simulink model "controle_v1"  (R2025b)
settings: Solver=FixedStepAuto  StartTime=0.0  StopTime=250  RelTol=1e-3
values from neighbouring files (symbols this model uses):
  Ta = 5    [controle_versao1.m]
  tao_1 = 60    [controle_versao1.m]
  tao_2 = 60    [controle_versao1.m]
  w1 = 0    [controle_versao1.m]
  w2 = 0    [controle_versao1.m]
  w3 = 0    [controle_versao1.m]
  w4 = 0    [controle_versao1.m]
undefined symbols (not defined in the file or in its folder): dspblkCoreblockFVToolHelper, gcbh, tao
libraries: dspobslib x1
settings Model: Creator=thoma  LastModifiedBy=thoma
settings ModelReferenceCC: EnableRefExpFcnMdlSchedulingChecks=on
settings RTWCC: GPUComputeCapability=3.5

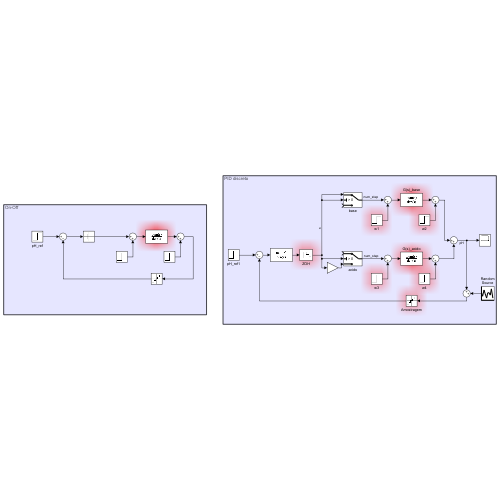
[thumbnail: Simulink's stored preview of the top-level diagram]
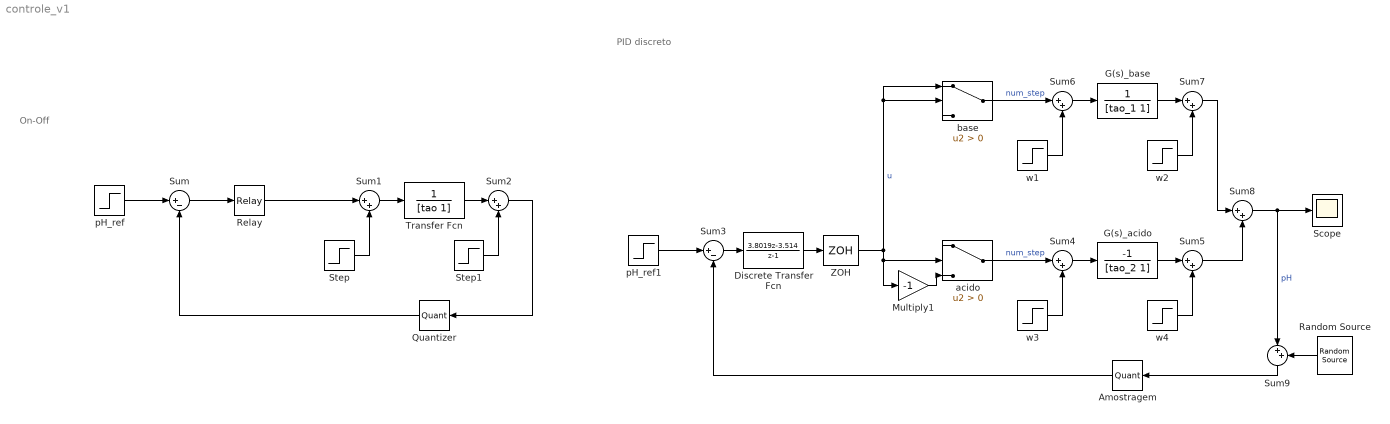
== system controle_v1 ==
  note: PID discreto
  note: On-Off
  Amostragem : Quantizer  QuantizationInterval=Ta
  Discrete Transfer Fcn : DiscreteTransferFcn  LoadFcn=dspblkCoreblockFVToolHelper(gcbh,'load');  Numerator=[3.8019 -3.514]  Denominator=[1 -1]  SampleTime=5
      settings: CopyFcn=dspblkCoreblockFVToolHelper(gcbh,'copy');  DeleteFcn=dspblkCoreblockFVToolHelper(gcbh,'close');  ModelCloseFcn=dspblkCoreblockFVToolHelper(gcbh,'close');  PreSaveFcn=dspblkCoreblockFVToolHelper(gcbh,'presave');  PostSaveFcn=dspblkCoreblockFVToolHelper(gcbh,'postsave');  CloseFcn=dspblkCoreblockFVToolHelper(gcbh,'close');
  G(s)_acido : TransferFcn  Numerator=[-1]  Denominator=[tao_2 1]
  G(s)_base : TransferFcn  Denominator=[tao_1 1]
  Multiply1 : Gain  Gain=-1
  Quantizer : Quantizer
  Random Source : dspobslib/Random Source  SrcType=Gaussian  NormMethod=Ziggurat  CltLength=12  MinVal=0  MaxVal=1  MeanVal=0  VarVal=1  RepMode=Not repeatable  rawSeed=1  IsInherit=off  SampMode=Continuous  SampTime=1  SampFrame=1  DataType=Double  OutComplex=Real  OutputFrames=off
  Relay : Relay  OnSwitchValue=3  OffSwitchValue=3  OnOutputValue=14
  Scope : Scope
      settings: ActiveDisplayYMinimum=-0.41212388639224318  ActiveDisplayYMaximum=3.7091149775301897
  Step : Step  SampleTime=0
  Step1 : Step  SampleTime=0
  Sum : Sum  Inputs=|+-
  Sum{1..2,4..9} (8 alike) : Sum  Inputs=|++
  Sum3 : Sum  Inputs=|+-
  Transfer Fcn : TransferFcn  Denominator=[tao 1]
  ZOH : ZeroOrderHold  SampleTime=Ta
  acido : Switch  Criteria=u2 > Threshold  SaturateOnIntegerOverflow=off  InputSameDT=off
  base : Switch  Criteria=u2 > Threshold  SaturateOnIntegerOverflow=off  InputSameDT=off
  pH_ref : Step  Time=0  After=3  SampleTime=0
  pH_ref1 : Step  Time=0  After=3  SampleTime=0
  w1 : Step  Time=0  After=w1  SampleTime=0
  w2 : Step  After=w2  SampleTime=0
  w3 : Step  After=w3  SampleTime=0
  w4 : Step  After=w4  SampleTime=0
  wires:
  Quantizer/1 -> Sum/2
  Sum1/1 -> Transfer Fcn/1
  Transfer Fcn/1 -> Sum2/1
  Sum2/1 -> Quantizer/1
  Step/1 -> Sum1/2
  Step1/1 -> Sum2/2
  Sum/1 -> Relay/1
  pH_ref/1 -> Sum/1
  Relay/1 -> Sum1/1
  Amostragem/1 -> Sum3/2
  Discrete Transfer Fcn/1 -> ZOH/1
  Sum4/1 -> G(s)_acido/1
  G(s)_acido/1 -> Sum5/1
  w4/1 -> Sum5/2
  w3/1 -> Sum4/2
  Sum3/1 -> Discrete Transfer Fcn/1
  pH_ref1/1 -> Sum3/1
  w1/1 -> Sum6/2
  Sum6/1 -> G(s)_base/1
  G(s)_base/1 -> Sum7/1
  w2/1 -> Sum7/2
  Sum5/1 -> Sum8/2
  Sum7/1 -> Sum8/1
  acido/1 -> Sum4/1  "num_step"
  base/1 -> Sum6/1  "num_step"
  ZOH/1 -> acido/2, Multiply1/1, base/1, base/2  "u"
  Multiply1/1 -> acido/3
  Sum9/1 -> Amostragem/1
  Sum8/1 -> Scope/1, Sum9/1  "pH"
  Random Source/1 -> Sum9/2
